simulink model "bot_motion"  (Simulink 6.4)
settings: Solver=ode45  StartTime=0.0  StopTime=10.0  RelTol=1e-3
StartFcn:
  | ppo_start
StopFcn:
  | ppo_stop
settings Model: LastModifiedBy=Raza

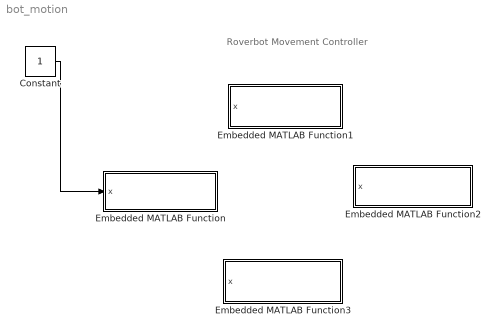
== system bot_motion ==
  note: Roverbot Movement Controller
  Constant : Constant  Value=1  OutDataType=sfix(16)  ConRadixGroup=Use specified scaling  OutScaling=2^0  SampleTime=inf  FramePeriod=inf
  Embedded MATLAB Function : Stateflow chart
  Embedded MATLAB Function1 : Stateflow chart
  Embedded MATLAB Function2 : Stateflow chart
  Embedded MATLAB Function3 : Stateflow chart
  wires:
  Constant/1 -> Embedded MATLAB Function/1(x)

== matlab function Embedded MATLAB Function1 ==
  data: x input inherited
function GoStraight(x)
MoveForward(x);

== matlab function Embedded MATLAB Function ==
  data: x input inherited
function GoLeft(x)
MoveLeft(x);

== matlab function Embedded MATLAB Function2 ==
  data: x input inherited
function GoRight(x)
MoveRight(x);

== matlab function Embedded MATLAB Function3 ==
  data: x input inherited
function GoBackwards(x)
MoveBackward(x);
